simulink model "linear_1_dof_1st_order"  (Simulink 7.7)
settings: Solver=ode45  StartTime=0.0  StopTime=50  RelTol=1e-4
values from neighbouring files (symbols this model uses):
  b_a = 1    [matlab_start.m]
  f_thresh = 1000    [matlab_start.m]
  gamma = 7    [matlab_start.m]
  k1 = 10    [matlab_start.m]
  k2 = 10    [matlab_start.m]
  k_a = 10    [matlab_start.m]
  kd = 0    [matlab_start.m]
  ki = 30.025    [matlab_start.m]
  kp = 0.15013    [matlab_start.m]
libraries: commnoisgen2 x1, mpclib x1
settings Model: Creator=mkillpack  LastModifiedBy=mkillpack
settings SolverCC: MaxConsecutiveMinStep=3  ZeroCrossAlgorithm=Adaptive
settings OptimizationCC: SimCompilerOptimization=On

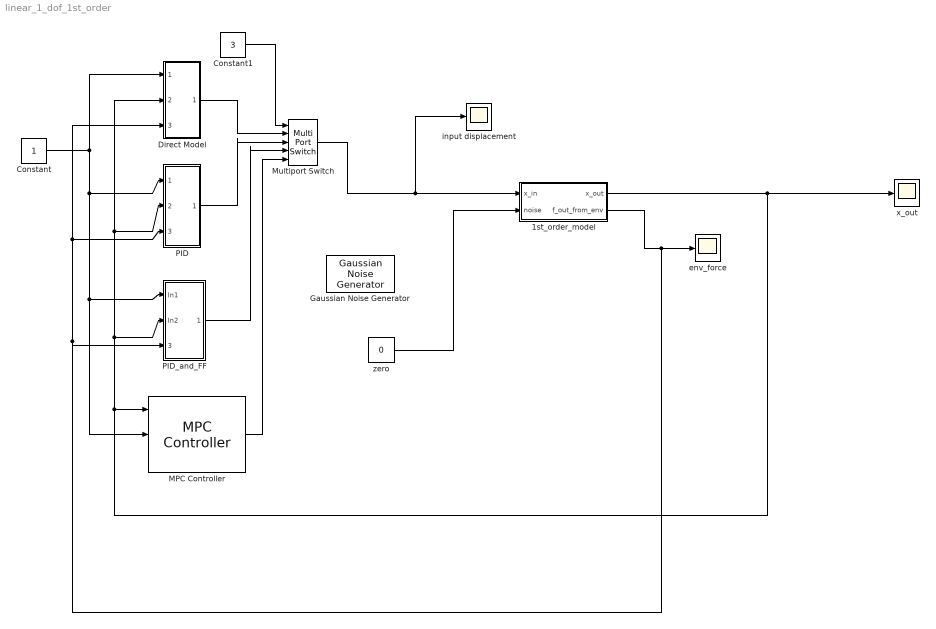
== system linear_1_dof_1st_order ==
  1st_order_model : Subsystem
  Constant : Constant
  Constant1 : Constant  Value=3
  Direct Model : Subsystem
  Gaussian Noise Generator : commnoisgen2/Gaussian Noise Generator  SystemSampleTime=-1  m=2  d=2  s=0  Ts=.01  frameBased=off  sampPerFrame=1  orient=off  outDataType=double
  MPC Controller : mpclib/MPC Controller  SystemSampleTime=-1  mpcobj=MPC1  n_mv=0  x0=[]  ref_from_ws=off  ref_signal_name=[]  ref_preview=on  md_from_ws=off  md_signal_name=[]  md_preview=on  from_project=off  md_inport=on  mv_inport=off  lims_inport=off  switch_inport=off  enable_value=0  project_file=MPCtask.mat  is_multiple=0  cost_outport=off  return_sequence=off
  Multiport Switch : MultiPortSwitch  Inputs=4  zeroidx=off
  PID : Subsystem
  PID_and_FF : Subsystem
  env_force : Scope
      settings: YMin=10.6  YMax=10.645  SaveName=ScopeData2
  input displacement : Scope
  x_out : Scope
      settings: YMin=0  YMax=2  SaveName=ScopeData3
  zero : Constant  Value=0
  wires:
  Constant1/1 -> Multiport Switch/1
  Multiport Switch/1 -> 1st_order_model/1(x_in), input displacement/1
  Direct Model/1(Out1) -> Multiport Switch/2
  PID/1(Out1) -> Multiport Switch/3
  PID_and_FF/1(Out1) -> Multiport Switch/4
  MPC Controller/1 -> Multiport Switch/5
  Constant/1 -> Direct Model/1(In1), PID/1(In1), MPC Controller/2, PID_and_FF/1(In1)
  1st_order_model/1(x_out) -> x_out/1, MPC Controller/1, PID_and_FF/2(In2), PID/2(In2), Direct Model/2(In2)
  1st_order_model/2(f_out_from_env) -> env_force/1, Direct Model/3(f_ext), PID/3(f_ext), PID_and_FF/3(f_ext)
  zero/1 -> 1st_order_model/2(noise)

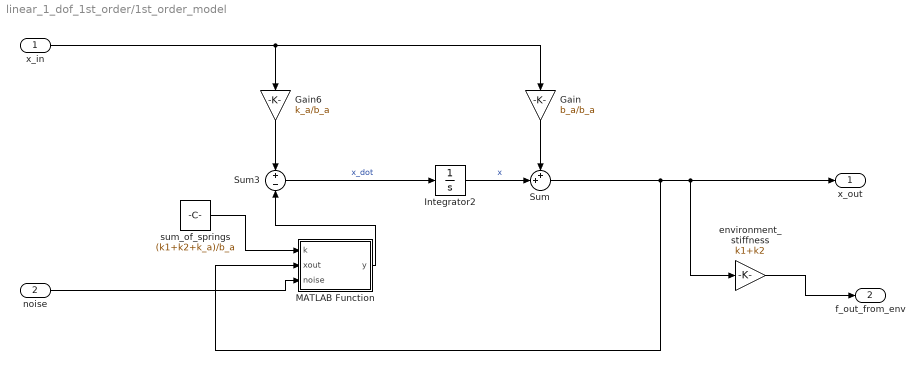
== system linear_1_dof_1st_order/1st_order_model ==
  x_in : Inport
  noise : Inport  Port=2
  Gain : Gain  Gain=b_a/b_a
  Gain6 : Gain  Gain=k_a/b_a
  Integrator2 : Integrator
  MATLAB Function : Stateflow chart  TreatAsAtomicUnit=on
  Sum : Sum  Inputs=++|
  Sum3 : Sum  Inputs=+|-
  environment_stiffness : Gain  Gain=k1+k2
  sum_of_springs : Constant  Value=(k1+k2+k_a)/b_a
  x_out : Outport
  f_out_from_env : Outport  Port=2
  wires:
  x_in/1 -> Gain6/1, Gain/1
  Sum/1 -> MATLAB Function/2(xout), x_out/1, environment_stiffness/1
  Sum3/1 -> Integrator2/1  "x_dot"
  MATLAB Function/1(y) -> Sum3/2
  Gain6/1 -> Sum3/1
  Gain/1 -> Sum/1
  Integrator2/1 -> Sum/2  "x"
  sum_of_springs/1 -> MATLAB Function/1(k)
  noise/1 -> MATLAB Function/3(noise)
  environment_stiffness/1 -> f_out_from_env/1

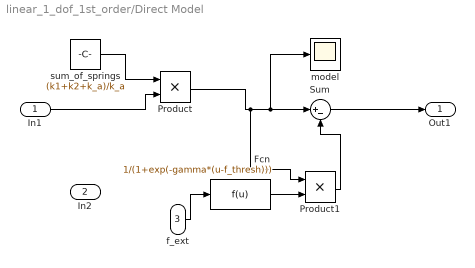
== system linear_1_dof_1st_order/Direct Model ==
  In1 : Inport
  In2 : Inport  Port=2
  f_ext : Inport  Port=3
  Fcn : Fcn  Expr=1/(1+exp(-gamma*(u-f_thresh)))
  Product : Product  RndMeth=Zero
  Product1 : Product  RndMeth=Zero
  Sum : Sum  Inputs=|+-
  model : Scope
      settings: YMin=0  YMax=1.5  SaveName=ScopeData4
  sum_of_springs : Constant  Value=(k1+k2+k_a)/k_a
  Out1 : Outport
  wires:
  In1/1 -> Product/2
  sum_of_springs/1 -> Product/1
  Product/1 -> Sum/1, model/1, Product1/1
  Sum/1 -> Out1/1
  f_ext/1 -> Fcn/1
  Fcn/1 -> Product1/2
  Product1/1 -> Sum/2

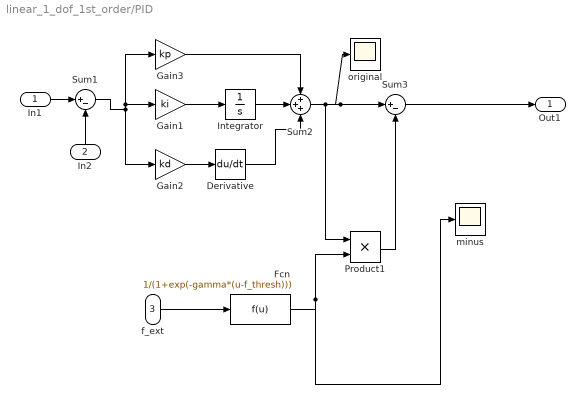
== system linear_1_dof_1st_order/PID ==
  In1 : Inport
  In2 : Inport  Port=2
  f_ext : Inport  Port=3
  Derivative : Derivative
  Fcn : Fcn  Expr=1/(1+exp(-gamma*(u-f_thresh)))
  Gain1 : Gain  Gain=ki
  Gain2 : Gain  Gain=kd
  Gain3 : Gain  Gain=kp
  Integrator : Integrator
  Product1 : Product  RndMeth=Zero
  Sum1 : Sum  Inputs=|+-
  Sum2 : Sum  Inputs=+++
  Sum3 : Sum  Inputs=|+-
  minus : Scope
      settings: YMin=6  YMax=25
  original : Scope
      settings: SaveName=ScopeData5
  Out1 : Outport
  wires:
  Gain2/1 -> Derivative/1
  Integrator/1 -> Sum2/2
  Derivative/1 -> Sum2/3
  Sum1/1 -> Gain2/1, Gain3/1, Gain1/1
  Gain3/1 -> Sum2/1
  Gain1/1 -> Integrator/1
  In2/1 -> Sum1/2
  In1/1 -> Sum1/1
  f_ext/1 -> Fcn/1
  Sum2/1 -> Product1/1, Sum3/1, original/1
  Sum3/1 -> Out1/1
  Fcn/1 -> Product1/2, minus/1
  Product1/1 -> Sum3/2

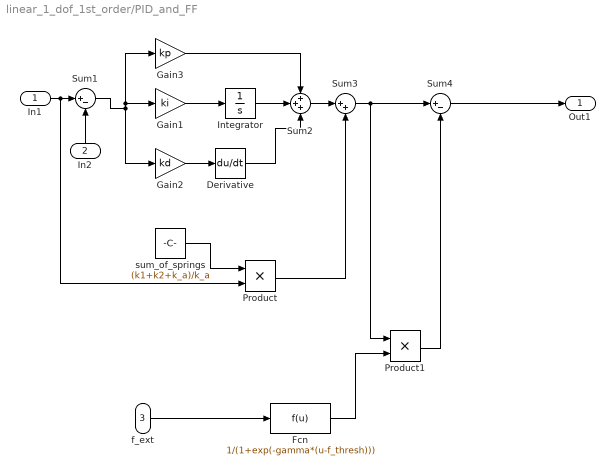
== system linear_1_dof_1st_order/PID_and_FF ==
  In1 : Inport
  In2 : Inport  Port=2
  f_ext : Inport  Port=3
  Derivative : Derivative
  Fcn : Fcn  Expr=1/(1+exp(-gamma*(u-f_thresh)))
  Gain1 : Gain  Gain=ki
  Gain2 : Gain  Gain=kd
  Gain3 : Gain  Gain=kp
  Integrator : Integrator
  Product : Product  RndMeth=Zero
  Product1 : Product  RndMeth=Zero
  Sum1 : Sum  Inputs=|+-
  Sum2 : Sum  Inputs=+++
  Sum3 : Sum  Inputs=|++
  Sum4 : Sum  Inputs=|+-
  sum_of_springs : Constant  Value=(k1+k2+k_a)/k_a
  Out1 : Outport
  wires:
  Gain2/1 -> Derivative/1
  Integrator/1 -> Sum2/2
  Derivative/1 -> Sum2/3
  Sum1/1 -> Gain2/1, Gain3/1, Gain1/1
  Gain3/1 -> Sum2/1
  Gain1/1 -> Integrator/1
  In2/1 -> Sum1/2
  In1/1 -> Sum1/1, Product/2
  Sum3/1 -> Product1/1, Sum4/1
  Sum2/1 -> Sum3/1
  sum_of_springs/1 -> Product/1
  Product/1 -> Sum3/2
  f_ext/1 -> Fcn/1
  Fcn/1 -> Product1/2
  Product1/1 -> Sum4/2
  Sum4/1 -> Out1/1

== matlab function 1st_order_model/MATLAB Function ==
  data: k input double; xout input double; y output double; noise input double
function y = fcn(k, xout, noise)
%#codegen

y = (k+noise)*xout;
